simulink model "DSimulator_robot1DOFV2"  (R2021a)
settings: Solver=ode1  StartTime=0.0  StopTime=10  FixedStep=0.001  RelTol=1e-3  EnableMultiTasking=on
values from neighbouring files (symbols this model uses):
  Tau = u(12)    [Dynamic_robot1DOFV.m]
undefined symbols (not defined in the file or in its folder): Dynamic_robot1DOFV, simpleRobotPlotv2
libraries: simulink x1
settings Model: Creator=E. Dean  LastModifiedBy=migue
settings SolverCC: AlgebraicLoopSolver=TrustRegion
settings DataIOCC: LimitDataPoints=on  SaveFormat=Array  SignalLoggingSaveFormat=ModelDataLogs  ReturnWorkspaceOutputs=off
settings OptimizationCC: ExpressionDepthLimit=2147483647  LifeSpan=inf
settings DebuggingCC: UnderspecifiedInitializationDetection=Classic  MergeDetectMultiDrivingBlocksExec=none  SolverPrmCheckMsg=warning  FcnCallInpInsideContextMsg=warning  StateNameClashWarn=warning  SFUnexpectedBacktrackingDiag=warning  SFNoUnconditionalDefaultTransitionDiag=warning  SFExecutionAtInitializationDiag=none  SFMachineParentedDataDiag=warning  ArithmeticOperatorsInVariantConditions=warning
settings HardwareCC: ProdBitPerPointer=32  ProdBitPerSizeT=32  ProdBitPerPtrDiffT=32  ProdLargestAtomicFloat=None  ProdIntDivRoundTo=Undefined  ProdEndianess=Unspecified  ProdWordSize=32  ProdHWDeviceType=32-bit Generic
settings ModelReferenceCC: PropagateSignalLabelsOutOfModel=off
settings SFSimCC: SimUseLocalCustomCode=off  CustomCodeUndefinedFunction=UseInterfaceOnly
settings RTWCC: RTWUseLocalCustomCode=off
settings CodeAppCC: StateflowObjectComments=on
settings GRTTargetCC: TargetLangStandard=C89/C90 (ANSI)  CombineOutputUpdateFcns=off  GRTInterface=on
settings ConfigComp: CovMetricSettings=dw  CovSaveCumulativeToWorkspaceVar=on  CovSaveSingleToWorkspaceVar=on

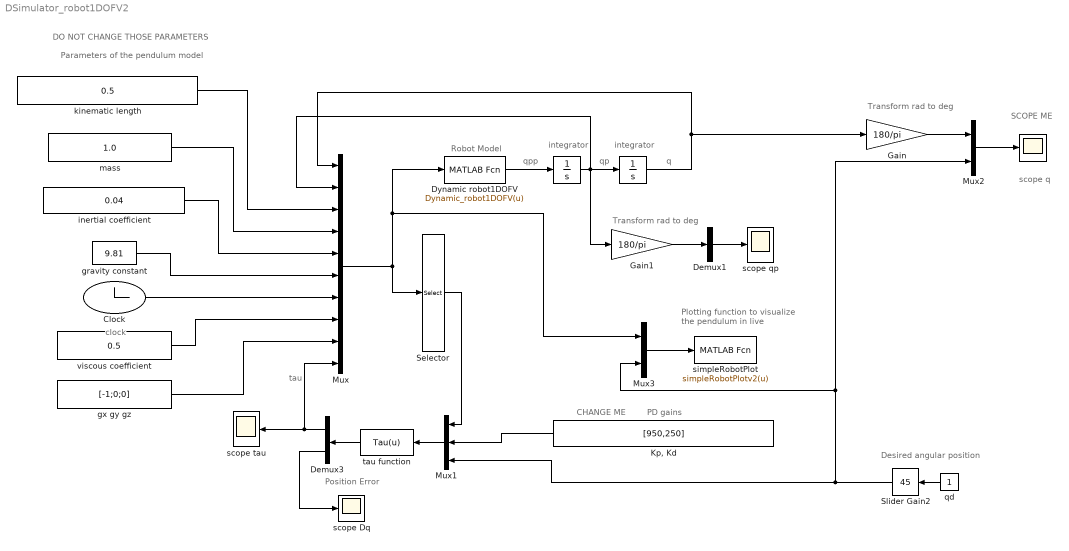
== system DSimulator_robot1DOFV2 ==
  note: SCOPE ME
  note: CHANGE ME
  note: q
  note: qp
  note: qpp
  note: tau
  note: DO NOT CHANGE THOSE PARAMETERS
  note: clock
  note: Parameters of the pendulum model
  note: Position Error
  note: scope q
  note: Transform rad to deg
  note: integrator
  note: integrator
  note: Robot Model
  note: Plotting function to
      | visualize the pendulum in live
  note: PD gains
  note: Desired angular position
  note: Transform rad to deg
  " " : Integrator  InitialCondition=[0]
  "  " : Integrator  InitialCondition=[0]
  "    " : Scope
  Clock : Clock
  Demux1 : Demux  Outputs=1
  Demux3 : Demux  Outputs=2
  Dynamic robot1DOFV : MATLABFcn  MATLABFcn=Dynamic_robot1DOFV(u)  OutputDimensions=1
  Gain : Gain  Gain=180/pi
  Gain1 : Gain  Gain=180/pi
  "Kp, Kd" : Constant  Value=[950,250]
  Mux : Mux  Inputs=10
  Mux1 : Mux  Inputs=3
  Mux2 : Mux  Inputs=2
  Mux3 : Mux  Inputs=2
  Selector : Selector  InputPortWidth=12  IndexOptions=Index vector (dialog)  Indices=[1:11]  OutputSizes=1
  Slider Gain2 : simulink/Math Operations/Slider Gain  gain=45  low=-90  high=90
  gravity constant : Constant  Value=9.81
  gx gy gz : Constant  Value=[-1;0;0]
  inertial coefficient : Constant  Value=0.04
  kinematic length : Constant  Value=0.5
  "mass " : Constant  Value=1.0
  qd : Constant
  scope Dq : Scope
  scope qp : Scope
  scope tau : Scope
  simpleRobotPlot : MATLABFcn  MATLABFcn=simpleRobotPlotv2(u)  OutputDimensions=0
  tau function : MATLABFcn  MATLABFcn=Tau(u)  OutputDimensions=2
  "viscous coefficient " : Constant  Value=0.5
  wires:
  " "/1 -> "  "/1, Gain1/1, Mux/2
  Mux/1 -> Selector/1, Dynamic robot1DOFV/1, Mux3/1
  Gain1/1 -> Demux1/1
  Demux1/1 -> scope qp/1
  kinematic length/1 -> Mux/3
  "mass "/1 -> Mux/4
  inertial coefficient/1 -> Mux/5
  gravity constant/1 -> Mux/6
  Clock/1 -> Mux/7
  "viscous coefficient "/1 -> Mux/8
  gx gy gz/1 -> Mux/9
  Mux1/1 -> tau function/1
  Selector/1 -> Mux1/1
  "Kp, Kd"/1 -> Mux1/2
  Slider Gain2/1 -> Mux2/2, Mux3/2, Mux1/3
  Dynamic robot1DOFV/1 -> " "/1
  tau function/1 -> Demux3/1
  Demux3/1 -> scope tau/1, Mux/10
  Demux3/2 -> scope Dq/1
  "  "/1 -> Mux/1, Gain/1
  Mux3/1 -> simpleRobotPlot/1
  Gain/1 -> Mux2/1
  Mux2/1 -> "    "/1
  qd/1 -> Slider Gain2/1
